simulink model "hw5_discrete_2dof"  (R2014b)
settings: Solver=ode45  StartTime=0.0  StopTime=10  RelTol=1e-3
values from neighbouring files (symbols this model uses):
  a1 = -2*cwh    [RST_hw4_fall18.m]    (also in hw5.m = -(1+exp(-hpt)); oscillator_RST.m)
  a2 = 1    [RST_hw4_fall18.m]    (also in hw5.m = exp(-hpt); oscillator_RST.m)
  b1 = 1-cwh    [RST_hw4_fall18.m]    (also in hw5.m = Km*tau*(hpt-1+exp(-hpt)); oscillator_RST.m)
  b2 = b1    [RST_hw4_fall18.m]    (also in hw5.m = Km*tau*(1-(1+hpt)*exp(-hpt)); oscillator_RST.m)
  ea = exp(h*a)    [hw5.m]
  h = findobj(gcf,'Type','line')    [AW_5_3.m]    (also in L4_RST_spring16.m = 0.1; PS4_ship_heading_RST_3h_script.m = 0.2; PS4_ship_heading_RST_noaa_script.m = 0.2; PS4_ship_heading_RST_script.m = 0.2)
  r1 = double(subs(sol.r1, vars, vals))    [AW_5_2.m]    (also in L4_RST_spring16.m = -0.856007930368168*a_d + 0.143992069631831; RST_example_spring18.m = params(1); hw5.m = -0.878368264722988*ea + 0.115597706410771)
  s0 = double(subs(sol.s0, vars, vals))    [AW_5_2.m]    (also in L4_RST_spring16.m = -28.7984139263664*a_d + 32.9380169529651; RST_example_spring18.m = params(2); hw5.m = -1.34327624390048*ea + 1.52396058689998)
  s1 = double(subs(sol.s1, vars, vals))    [AW_5_2.m]    (also in L4_RST_spring16.m = 24.6588108997672*a_d - 28.7984139263663; RST_example_spring18.m = params(3); hw5.m = 0.972399357505391*ea - 1.15308370050492)
  t0 = subs(Acs, z, 1) / subs(Bsa, z, 1)    [AW_5_3.m]    (also in L4_RST_spring16.m = 4.1396030266; RST_example_spring18.m = 0.210526315789; RST_sym.m = subs(Ac, z, 1) / subs(B, z, 1); RST_sym_handout.m = subs(Ac, z, 1) / subs(B, z, 1))
settings Model: Creator=kjartan  LastModifiedBy=kjartan

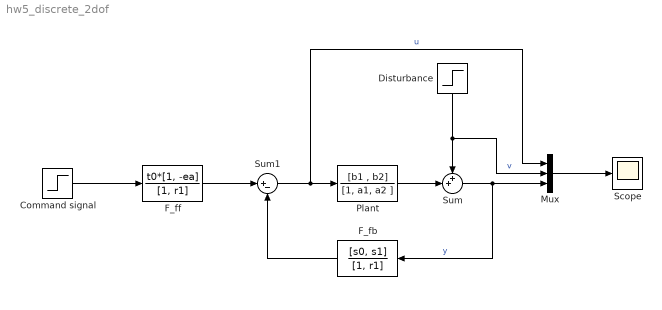
== system hw5_discrete_2dof ==
  Command signal : Step  Time=0  SampleTime=0
  Disturbance : Step  Time=5  SampleTime=0
  F_fb : DiscreteTransferFcn  Numerator=[s0, s1]  Denominator=[1, r1]  SampleTime=h
  F_ff : DiscreteTransferFcn  Numerator=t0*[1, -ea]  Denominator=[1, r1]  SampleTime=h
  Mux : Mux  Inputs=3
  Plant : DiscreteTransferFcn  Numerator=[b1 , b2]  Denominator=[1, a1, a2 ]  SampleTime=h
  Scope : Scope
      settings: ShowLegends=on
  Sum : Sum  Inputs=++|
  Sum1 : Sum  Inputs=|+-
  wires:
  Sum/1 -> F_fb/1, Mux/3  "y"
  Plant/1 -> Sum/2
  Mux/1 -> Scope/1
  Command signal/1 -> F_ff/1
  Disturbance/1 -> Mux/2, Sum/1  "v"
  Sum1/1 -> Plant/1, Mux/1  "u"
  F_fb/1 -> Sum1/2
  F_ff/1 -> Sum1/1
